simulink model "problem2"  (R2020a)
settings: Solver=VariableStepAuto  StartTime=0.0  StopTime=10.0  RelTol=1e-3
values from neighbouring files (symbols this model uses):
  b = 350.0    [problem2_data.sldd]
  K1 = 80000.0    [problem2_data.sldd]
  K2 = 500000.0    [problem2_data.sldd]
  M1 = 2500.0    [problem2_data.sldd]
  M2 = 320.0    [problem2_data.sldd]
settings Model: Creator=USER  LastModifiedBy=USER

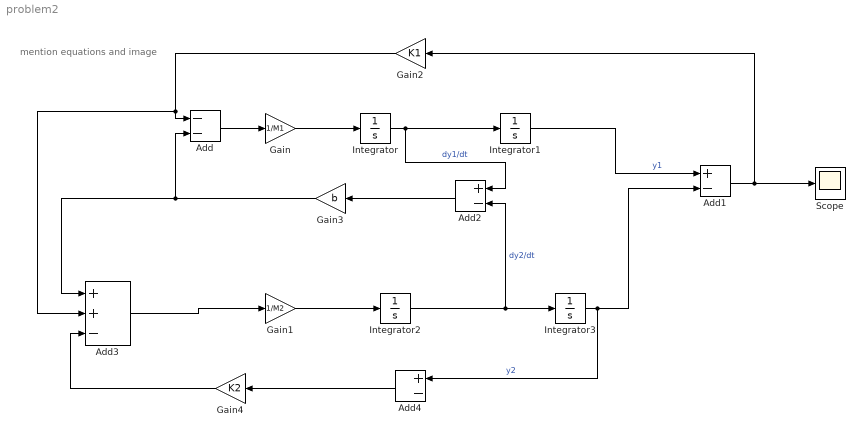
== system problem2 ==
  note: mention equations and image
  Add : Sum  Inputs=--
  Add1 : Sum  Inputs=+-
  Add2 : Sum  Inputs=+-
  Add3 : Sum  Inputs=++-
  Add4 : Sum  Inputs=+-
  Gain : Gain  Gain=1/M1
  Gain1 : Gain  Gain=1/M2
  Gain2 : Gain  Gain=K1
  Gain3 : Gain  Gain=b
  Gain4 : Gain  Gain=K2
  Integrator{,1..3} (4 alike) : Integrator
  Scope : Scope
  wires:
  Integrator1/1 -> Add1/1  "y1"
  Integrator/1 -> Add2/1, Integrator1/1  "dy1/dt"
  Add4/1 -> Gain4/1
  ? -> Add4/2
  Add1/1 -> Gain2/1, Scope/1
  Gain2/1 -> Add3/2, Add/1
  Add/1 -> Gain/1
  Gain1/1 -> Integrator2/1
  Gain3/1 -> Add3/1, Add/2
  Gain4/1 -> Add3/3
  Add2/1 -> Gain3/1
  Integrator2/1 -> Add2/2, Integrator3/1  "dy2/dt"
  Integrator3/1 -> Add4/1, Add1/2  "y2"
  Gain/1 -> Integrator/1
  Add3/1 -> Gain1/1
